simulink model "ADAC_AEBS_FailOperationTest_A2_cs"  (Simulink 7.6)
settings: Solver=ode5  SolverMode=SingleTasking  StartTime=0.0  StopTime=inf  FixedStep=1/100  RelTol=1e-3
PreLoadFcn:
  | check_NUTS_defined;
  | 
  | assignin('base',['model_closed_' bdroot],false);addpath('../includes_AEBS');
InitFcn:
  | PreScanExperimentInitFcn(bdroot)
StopFcn:
  | PreScanExperimentStopFcn(bdroot)
undefined symbols (not defined in the file): DiscIntNeverNeededParam, x_ini_VRML, y_ini_VRML, z_ini_VRML
libraries: simulink x25, PreScanSimulinkLibrary x12, simulink_extras x8, PreScanUsefulBlocks x5, simulink_need_slupdate x1
(part 4 of 7)

== system ADAC_AEBS_FailOperationTest_A2_cs/VISULightSource_Audi_A8_1/conv_FogLightFrontRight ==
  on_off : Inport
  OffColor : Constant  Value="[51   51   51  255   77   77   77  255  102  102  102  255    0    0    0  255]"
  OnColor : Constant  Value="[51   51   51  255  204  204  204  255  102  102  102  255  510  510  510  255]"
  Switch1 : Switch  Threshold=0.5
  RGBcolor : Outport
  wires:
  OffColor/1 -> Switch1/3  "off"
  OnColor/1 -> Switch1/1  "on"
  on_off/1 -> Switch1/2
  Switch1/1 -> RGBcolor/1

== system ADAC_AEBS_FailOperationTest_A2_cs/VISULightSource_Audi_A8_1/conv_FogLightRearLeft ==
  on_off : Inport
  OffColor : Constant  Value="[51   51   51  255   92    0    0  255  102  102  102  255    0    0    0  255]"
  OnColor : Constant  Value="[51   51   51  255  332   51    0  255  102  102  102  255  583   10    0  255]"
  Switch1 : Switch  Threshold=0.5
  RGBcolor : Outport
  wires:
  OffColor/1 -> Switch1/3  "off"
  OnColor/1 -> Switch1/1  "on"
  on_off/1 -> Switch1/2
  Switch1/1 -> RGBcolor/1

== system ADAC_AEBS_FailOperationTest_A2_cs/VISULightSource_Audi_A8_1/conv_FogLightRearRight ==
  on_off : Inport
  OffColor : Constant  Value="[51   51   51  255   92    0    0  255  102  102  102  255    0    0    0  255]"
  OnColor : Constant  Value="[51   51   51  255  332   51    0  255  102  102  102  255  583   10    0  255]"
  Switch1 : Switch  Threshold=0.5
  RGBcolor : Outport
  wires:
  OffColor/1 -> Switch1/3  "off"
  OnColor/1 -> Switch1/1  "on"
  on_off/1 -> Switch1/2
  Switch1/1 -> RGBcolor/1

== system ADAC_AEBS_FailOperationTest_A2_cs/VISULightSource_Audi_A8_1/conv_IndicatorLightsLeft ==
  on_off : Inport
  OffColor : Constant  Value="[51   51   51  255  138   69    0  255  102  102  102  255    0    0    0  255]"
  OnColor : Constant  Value="[51   51   51  255  255  128    0  255  102  102  102  255  255  191    0  255]"
  Switch1 : Switch  Threshold=0.5
  RGBcolor : Outport
  wires:
  Switch1/1 -> RGBcolor/1
  on_off/1 -> Switch1/2
  OnColor/1 -> Switch1/1  "on"
  OffColor/1 -> Switch1/3  "off"

== system ADAC_AEBS_FailOperationTest_A2_cs/VISULightSource_Audi_A8_1/conv_IndicatorLightsRight ==
  on_off : Inport
  OffColor : Constant  Value="[51   51   51  255  138   69    0  255  102  102  102  255    0    0    0  255]"
  OnColor : Constant  Value="[51   51   51  255  255  128    0  255  102  102  102  255  255  191    0  255]"
  Switch1 : Switch  Threshold=0.5
  RGBcolor : Outport
  wires:
  OffColor/1 -> Switch1/3  "off"
  OnColor/1 -> Switch1/1  "on"
  on_off/1 -> Switch1/2
  Switch1/1 -> RGBcolor/1

== system ADAC_AEBS_FailOperationTest_A2_cs/VISULightSource_Audi_A8_1/conv_MainLightFrontLeft ==
  on_off : Inport
  OffColor : Constant  Value="[26   26   26  255   77   77   77  255  102  102  102  255    0    0    0  255]"
  OnColor : Constant  Value="[51   51   51  255  255  255  255  255  102  102  102  255  683  683  683  255]"
  Switch1 : Switch  Threshold=0.5
  RGBcolor : Outport
  wires:
  OffColor/1 -> Switch1/3  "off"
  OnColor/1 -> Switch1/1  "on"
  on_off/1 -> Switch1/2
  Switch1/1 -> RGBcolor/1

== system ADAC_AEBS_FailOperationTest_A2_cs/VISULightSource_Audi_A8_1/conv_MainLightFrontRight ==
  on_off : Inport
  OffColor : Constant  Value="[26   26   26  255   77   77   77  255  102  102  102  255    0    0    0  255]"
  OnColor : Constant  Value="[51   51   51  255  255  255  255  255  102  102  102  255  683  683  683  255]"
  Switch1 : Switch  Threshold=0.5
  RGBcolor : Outport
  wires:
  OffColor/1 -> Switch1/3  "off"
  OnColor/1 -> Switch1/1  "on"
  on_off/1 -> Switch1/2
  Switch1/1 -> RGBcolor/1

== system ADAC_AEBS_FailOperationTest_A2_cs/VISULightSource_Audi_A8_1/conv_MainLightRearLeft ==
  on_off : Inport
  OffColor : Constant  Value="[51   51   51  255   92    0    0  255  102  102  102  255    0    0    0  255]"
  OnColor : Constant  Value="[51   51   51  255  322   51    0  255  102  102  102  255  255   40    0  255]"
  Switch1 : Switch  Threshold=0.5
  RGBcolor : Outport
  wires:
  OffColor/1 -> Switch1/3  "off"
  OnColor/1 -> Switch1/1  "on"
  on_off/1 -> Switch1/2
  Switch1/1 -> RGBcolor/1

== system ADAC_AEBS_FailOperationTest_A2_cs/VISULightSource_Audi_A8_1/conv_MainLightRearRight ==
  on_off : Inport
  OffColor : Constant  Value="[51   51   51  255   92    0    0  255  102  102  102  255    0    0    0  255]"
  OnColor : Constant  Value="[51   51   51  255  322   51    0  255  102  102  102  255  255   40    0  255]"
  Switch1 : Switch  Threshold=0.5
  RGBcolor : Outport
  wires:
  OffColor/1 -> Switch1/3  "off"
  OnColor/1 -> Switch1/1  "on"
  on_off/1 -> Switch1/2
  Switch1/1 -> RGBcolor/1

== system ADAC_AEBS_FailOperationTest_A2_cs/VISULightSource_Audi_A8_1/visu_BrakeLightLeft_0 ==
  Y : Inport
  Assignment : Assignment  IndexMode=Zero-based  SampleTime=TimeStep  IndexOptions=Starting index (dialog)  Indices=PortIndex  OutputSizes=[1 1]
  Data Store Read : DataStoreRead  DataStoreName=SimCoreActuators  SampleTime=TimeStep
  Data Store Write : DataStoreWrite  DataStoreName=SimCoreActuators
  wires:
  Y/1 -> Assignment/2
  Data Store Read/1 -> Assignment/1
  Assignment/1 -> Data Store Write/1

== system ADAC_AEBS_FailOperationTest_A2_cs/VISULightSource_Audi_A8_1/visu_BrakeLightRight_0 ==
  Y : Inport
  Assignment : Assignment  IndexMode=Zero-based  SampleTime=TimeStep  IndexOptions=Starting index (dialog)  Indices=PortIndex  OutputSizes=[1 1]
  Data Store Read : DataStoreRead  DataStoreName=SimCoreActuators  SampleTime=TimeStep
  Data Store Write : DataStoreWrite  DataStoreName=SimCoreActuators
  wires:
  Y/1 -> Assignment/2
  Data Store Read/1 -> Assignment/1
  Assignment/1 -> Data Store Write/1

== system ADAC_AEBS_FailOperationTest_A2_cs/VISULightSource_Audi_A8_1/visu_FogLightFrontLeft_0 ==
  Y : Inport
  Assignment : Assignment  IndexMode=Zero-based  SampleTime=TimeStep  IndexOptions=Starting index (dialog)  Indices=PortIndex  OutputSizes=[1 1]
  Data Store Read : DataStoreRead  DataStoreName=SimCoreActuators  SampleTime=TimeStep
  Data Store Write : DataStoreWrite  DataStoreName=SimCoreActuators
  wires:
  Y/1 -> Assignment/2
  Data Store Read/1 -> Assignment/1
  Assignment/1 -> Data Store Write/1

== system ADAC_AEBS_FailOperationTest_A2_cs/VISULightSource_Audi_A8_1/visu_FogLightFrontRight_0 ==
  Y : Inport
  Assignment : Assignment  IndexMode=Zero-based  SampleTime=TimeStep  IndexOptions=Starting index (dialog)  Indices=PortIndex  OutputSizes=[1 1]
  Data Store Read : DataStoreRead  DataStoreName=SimCoreActuators  SampleTime=TimeStep
  Data Store Write : DataStoreWrite  DataStoreName=SimCoreActuators
  wires:
  Y/1 -> Assignment/2
  Data Store Read/1 -> Assignment/1
  Assignment/1 -> Data Store Write/1

== system ADAC_AEBS_FailOperationTest_A2_cs/VISULightSource_Audi_A8_1/visu_FogLightRearLeft_0 ==
  Y : Inport
  Assignment : Assignment  IndexMode=Zero-based  SampleTime=TimeStep  IndexOptions=Starting index (dialog)  Indices=PortIndex  OutputSizes=[1 1]
  Data Store Read : DataStoreRead  DataStoreName=SimCoreActuators  SampleTime=TimeStep
  Data Store Write : DataStoreWrite  DataStoreName=SimCoreActuators
  wires:
  Y/1 -> Assignment/2
  Data Store Read/1 -> Assignment/1
  Assignment/1 -> Data Store Write/1

== system ADAC_AEBS_FailOperationTest_A2_cs/VISULightSource_Audi_A8_1/visu_FogLightRearRight_0 ==
  Y : Inport
  Assignment : Assignment  IndexMode=Zero-based  SampleTime=TimeStep  IndexOptions=Starting index (dialog)  Indices=PortIndex  OutputSizes=[1 1]
  Data Store Read : DataStoreRead  DataStoreName=SimCoreActuators  SampleTime=TimeStep
  Data Store Write : DataStoreWrite  DataStoreName=SimCoreActuators
  wires:
  Y/1 -> Assignment/2
  Data Store Read/1 -> Assignment/1
  Assignment/1 -> Data Store Write/1

== system ADAC_AEBS_FailOperationTest_A2_cs/VISULightSource_Audi_A8_1/visu_IndicatorLightsLeft_0 ==
  Y : Inport
  Assignment : Assignment  IndexMode=Zero-based  SampleTime=TimeStep  IndexOptions=Starting index (dialog)  Indices=PortIndex  OutputSizes=[1 1]
  Data Store Read : DataStoreRead  DataStoreName=SimCoreActuators  SampleTime=TimeStep
  Data Store Write : DataStoreWrite  DataStoreName=SimCoreActuators
  wires:
  Assignment/1 -> Data Store Write/1
  Data Store Read/1 -> Assignment/1
  Y/1 -> Assignment/2

== system ADAC_AEBS_FailOperationTest_A2_cs/VISULightSource_Audi_A8_1/visu_IndicatorLightsRight_0 ==
  Y : Inport
  Assignment : Assignment  IndexMode=Zero-based  SampleTime=TimeStep  IndexOptions=Starting index (dialog)  Indices=PortIndex  OutputSizes=[1 1]
  Data Store Read : DataStoreRead  DataStoreName=SimCoreActuators  SampleTime=TimeStep
  Data Store Write : DataStoreWrite  DataStoreName=SimCoreActuators
  wires:
  Y/1 -> Assignment/2
  Data Store Read/1 -> Assignment/1
  Assignment/1 -> Data Store Write/1

== system ADAC_AEBS_FailOperationTest_A2_cs/VISULightSource_Audi_A8_1/visu_MainLightFrontLeft_0 ==
  Y : Inport
  Assignment : Assignment  IndexMode=Zero-based  SampleTime=TimeStep  IndexOptions=Starting index (dialog)  Indices=PortIndex  OutputSizes=[1 1]
  Data Store Read : DataStoreRead  DataStoreName=SimCoreActuators  SampleTime=TimeStep
  Data Store Write : DataStoreWrite  DataStoreName=SimCoreActuators
  wires:
  Y/1 -> Assignment/2
  Data Store Read/1 -> Assignment/1
  Assignment/1 -> Data Store Write/1

== system ADAC_AEBS_FailOperationTest_A2_cs/VISULightSource_Audi_A8_1/visu_MainLightFrontRight_0 ==
  Y : Inport
  Assignment : Assignment  IndexMode=Zero-based  SampleTime=TimeStep  IndexOptions=Starting index (dialog)  Indices=PortIndex  OutputSizes=[1 1]
  Data Store Read : DataStoreRead  DataStoreName=SimCoreActuators  SampleTime=TimeStep
  Data Store Write : DataStoreWrite  DataStoreName=SimCoreActuators
  wires:
  Y/1 -> Assignment/2
  Data Store Read/1 -> Assignment/1
  Assignment/1 -> Data Store Write/1

== system ADAC_AEBS_FailOperationTest_A2_cs/VISULightSource_Audi_A8_1/visu_MainLightRearLeft_0 ==
  Y : Inport
  Assignment : Assignment  IndexMode=Zero-based  SampleTime=TimeStep  IndexOptions=Starting index (dialog)  Indices=PortIndex  OutputSizes=[1 1]
  Data Store Read : DataStoreRead  DataStoreName=SimCoreActuators  SampleTime=TimeStep
  Data Store Write : DataStoreWrite  DataStoreName=SimCoreActuators
  wires:
  Y/1 -> Assignment/2
  Data Store Read/1 -> Assignment/1
  Assignment/1 -> Data Store Write/1

== system ADAC_AEBS_FailOperationTest_A2_cs/VISULightSource_Audi_A8_1/visu_MainLightRearRight_0 ==
  Y : Inport
  Assignment : Assignment  IndexMode=Zero-based  SampleTime=TimeStep  IndexOptions=Starting index (dialog)  Indices=PortIndex  OutputSizes=[1 1]
  Data Store Read : DataStoreRead  DataStoreName=SimCoreActuators  SampleTime=TimeStep
  Data Store Write : DataStoreWrite  DataStoreName=SimCoreActuators
  wires:
  Y/1 -> Assignment/2
  Data Store Read/1 -> Assignment/1
  Assignment/1 -> Data Store Write/1

== system ADAC_AEBS_FailOperationTest_A2_cs/VISULightSource_Citroen_C3_1/conv_BrakeLightLeft ==
  on_off : Inport
  OffColor : Constant  Value="[51   51   51  255   92    0    0  255  102  102  102  255    0    0    0  255]"
  OnColor : Constant  Value="[51   51   51  255  332   51    0  255  102  102  102  255  583   47    0  255]"
  Switch1 : Switch  Threshold=0.5
  RGBcolor : Outport
  wires:
  OffColor/1 -> Switch1/3  "off"
  OnColor/1 -> Switch1/1  "on"
  on_off/1 -> Switch1/2
  Switch1/1 -> RGBcolor/1

== system ADAC_AEBS_FailOperationTest_A2_cs/VISULightSource_Citroen_C3_1/conv_BrakeLightRight ==
  on_off : Inport
  OffColor : Constant  Value="[51   51   51  255   92    0    0  255  102  102  102  255    0    0    0  255]"
  OnColor : Constant  Value="[51   51   51  255  332   51    0  255  102  102  102  255  583   47    0  255]"
  Switch1 : Switch  Threshold=0.5
  RGBcolor : Outport
  wires:
  OffColor/1 -> Switch1/3  "off"
  OnColor/1 -> Switch1/1  "on"
  on_off/1 -> Switch1/2
  Switch1/1 -> RGBcolor/1

== system ADAC_AEBS_FailOperationTest_A2_cs/VISULightSource_Citroen_C3_1/conv_FogLightFrontLeft ==
  on_off : Inport
  OffColor : Constant  Value="[51   51   51  255   77   77   77  255  102  102  102  255    0    0    0  255]"
  OnColor : Constant  Value="[51   51   51  255  204  204  204  255  102  102  102  255  510  510  510  255]"
  Switch1 : Switch  Threshold=0.5
  RGBcolor : Outport
  wires:
  OffColor/1 -> Switch1/3  "off"
  OnColor/1 -> Switch1/1  "on"
  on_off/1 -> Switch1/2
  Switch1/1 -> RGBcolor/1

== system ADAC_AEBS_FailOperationTest_A2_cs/VISULightSource_Citroen_C3_1/conv_FogLightFrontRight ==
  on_off : Inport
  OffColor : Constant  Value="[51   51   51  255   77   77   77  255  102  102  102  255    0    0    0  255]"
  OnColor : Constant  Value="[51   51   51  255  204  204  204  255  102  102  102  255  510  510  510  255]"
  Switch1 : Switch  Threshold=0.5
  RGBcolor : Outport
  wires:
  OffColor/1 -> Switch1/3  "off"
  OnColor/1 -> Switch1/1  "on"
  on_off/1 -> Switch1/2
  Switch1/1 -> RGBcolor/1

== system ADAC_AEBS_FailOperationTest_A2_cs/VISULightSource_Citroen_C3_1/conv_IndicatorLightsLeft ==
  on_off : Inport
  OffColor : Constant  Value="[51   51   51  255  138   69    0  255  102  102  102  255    0    0    0  255]"
  OnColor : Constant  Value="[51   51   51  255  255  128    0  255  102  102  102  255  255  191    0  255]"
  Switch1 : Switch  Threshold=0.5
  RGBcolor : Outport
  wires:
  Switch1/1 -> RGBcolor/1
  on_off/1 -> Switch1/2
  OnColor/1 -> Switch1/1  "on"
  OffColor/1 -> Switch1/3  "off"

== system ADAC_AEBS_FailOperationTest_A2_cs/VISULightSource_Citroen_C3_1/conv_IndicatorLightsRight ==
  on_off : Inport
  OffColor : Constant  Value="[51   51   51  255  138   69    0  255  102  102  102  255    0    0    0  255]"
  OnColor : Constant  Value="[51   51   51  255  255  128    0  255  102  102  102  255  255  191    0  255]"
  Switch1 : Switch  Threshold=0.5
  RGBcolor : Outport
  wires:
  OffColor/1 -> Switch1/3  "off"
  OnColor/1 -> Switch1/1  "on"
  on_off/1 -> Switch1/2
  Switch1/1 -> RGBcolor/1

== system ADAC_AEBS_FailOperationTest_A2_cs/VISULightSource_Citroen_C3_1/conv_MainLightFrontLeft ==
  on_off : Inport
  OffColor : Constant  Value="[26   26   26  255   77   77   77  255  102  102  102  255    0    0    0  255]"
  OnColor : Constant  Value="[51   51   51  255  255  255  255  255  102  102  102  255  683  683  683  255]"
  Switch1 : Switch  Threshold=0.5
  RGBcolor : Outport
  wires:
  OffColor/1 -> Switch1/3  "off"
  OnColor/1 -> Switch1/1  "on"
  on_off/1 -> Switch1/2
  Switch1/1 -> RGBcolor/1

== system ADAC_AEBS_FailOperationTest_A2_cs/VISULightSource_Citroen_C3_1/conv_MainLightFrontRight ==
  on_off : Inport
  OffColor : Constant  Value="[26   26   26  255   77   77   77  255  102  102  102  255    0    0    0  255]"
  OnColor : Constant  Value="[51   51   51  255  255  255  255  255  102  102  102  255  683  683  683  255]"
  Switch1 : Switch  Threshold=0.5
  RGBcolor : Outport
  wires:
  OffColor/1 -> Switch1/3  "off"
  OnColor/1 -> Switch1/1  "on"
  on_off/1 -> Switch1/2
  Switch1/1 -> RGBcolor/1

== system ADAC_AEBS_FailOperationTest_A2_cs/VISULightSource_Citroen_C3_1/conv_MainLightRearLeft ==
  on_off : Inport
  OffColor : Constant  Value="[51   51   51  255   92    0    0  255  102  102  102  255    0    0    0  255]"
  OnColor : Constant  Value="[51   51   51  255  322   51    0  255  102  102  102  255  255   40    0  255]"
  Switch1 : Switch  Threshold=0.5
  RGBcolor : Outport
  wires:
  OffColor/1 -> Switch1/3  "off"
  OnColor/1 -> Switch1/1  "on"
  on_off/1 -> Switch1/2
  Switch1/1 -> RGBcolor/1

== system ADAC_AEBS_FailOperationTest_A2_cs/VISULightSource_Citroen_C3_1/conv_MainLightRearRight ==
  on_off : Inport
  OffColor : Constant  Value="[51   51   51  255   92    0    0  255  102  102  102  255    0    0    0  255]"
  OnColor : Constant  Value="[51   51   51  255  322   51    0  255  102  102  102  255  255   40    0  255]"
  Switch1 : Switch  Threshold=0.5
  RGBcolor : Outport
  wires:
  OffColor/1 -> Switch1/3  "off"
  OnColor/1 -> Switch1/1  "on"
  on_off/1 -> Switch1/2
  Switch1/1 -> RGBcolor/1

== system ADAC_AEBS_FailOperationTest_A2_cs/VISULightSource_Citroen_C3_1/visu_BrakeLightLeft_0 ==
  Y : Inport
  Assignment : Assignment  IndexMode=Zero-based  SampleTime=TimeStep  IndexOptions=Starting index (dialog)  Indices=PortIndex  OutputSizes=[1 1]
  Data Store Read : DataStoreRead  DataStoreName=SimCoreActuators  SampleTime=TimeStep
  Data Store Write : DataStoreWrite  DataStoreName=SimCoreActuators
  wires:
  Y/1 -> Assignment/2
  Data Store Read/1 -> Assignment/1
  Assignment/1 -> Data Store Write/1

== system ADAC_AEBS_FailOperationTest_A2_cs/VISULightSource_Citroen_C3_1/visu_BrakeLightRight_0 ==
  Y : Inport
  Assignment : Assignment  IndexMode=Zero-based  SampleTime=TimeStep  IndexOptions=Starting index (dialog)  Indices=PortIndex  OutputSizes=[1 1]
  Data Store Read : DataStoreRead  DataStoreName=SimCoreActuators  SampleTime=TimeStep
  Data Store Write : DataStoreWrite  DataStoreName=SimCoreActuators
  wires:
  Y/1 -> Assignment/2
  Data Store Read/1 -> Assignment/1
  Assignment/1 -> Data Store Write/1

== system ADAC_AEBS_FailOperationTest_A2_cs/VISULightSource_Citroen_C3_1/visu_FogLightFrontLeft_0 ==
  Y : Inport
  Assignment : Assignment  IndexMode=Zero-based  SampleTime=TimeStep  IndexOptions=Starting index (dialog)  Indices=PortIndex  OutputSizes=[1 1]
  Data Store Read : DataStoreRead  DataStoreName=SimCoreActuators  SampleTime=TimeStep
  Data Store Write : DataStoreWrite  DataStoreName=SimCoreActuators
  wires:
  Y/1 -> Assignment/2
  Data Store Read/1 -> Assignment/1
  Assignment/1 -> Data Store Write/1

== system ADAC_AEBS_FailOperationTest_A2_cs/VISULightSource_Citroen_C3_1/visu_FogLightFrontRight_0 ==
  Y : Inport
  Assignment : Assignment  IndexMode=Zero-based  SampleTime=TimeStep  IndexOptions=Starting index (dialog)  Indices=PortIndex  OutputSizes=[1 1]
  Data Store Read : DataStoreRead  DataStoreName=SimCoreActuators  SampleTime=TimeStep
  Data Store Write : DataStoreWrite  DataStoreName=SimCoreActuators
  wires:
  Y/1 -> Assignment/2
  Data Store Read/1 -> Assignment/1
  Assignment/1 -> Data Store Write/1

== system ADAC_AEBS_FailOperationTest_A2_cs/VISULightSource_Citroen_C3_1/visu_IndicatorLightsLeft_0 ==
  Y : Inport
  Assignment : Assignment  IndexMode=Zero-based  SampleTime=TimeStep  IndexOptions=Starting index (dialog)  Indices=PortIndex  OutputSizes=[1 1]
  Data Store Read : DataStoreRead  DataStoreName=SimCoreActuators  SampleTime=TimeStep
  Data Store Write : DataStoreWrite  DataStoreName=SimCoreActuators
  wires:
  Assignment/1 -> Data Store Write/1
  Data Store Read/1 -> Assignment/1
  Y/1 -> Assignment/2

== system ADAC_AEBS_FailOperationTest_A2_cs/VISULightSource_Citroen_C3_1/visu_IndicatorLightsRight_0 ==
  Y : Inport
  Assignment : Assignment  IndexMode=Zero-based  SampleTime=TimeStep  IndexOptions=Starting index (dialog)  Indices=PortIndex  OutputSizes=[1 1]
  Data Store Read : DataStoreRead  DataStoreName=SimCoreActuators  SampleTime=TimeStep
  Data Store Write : DataStoreWrite  DataStoreName=SimCoreActuators
  wires:
  Y/1 -> Assignment/2
  Data Store Read/1 -> Assignment/1
  Assignment/1 -> Data Store Write/1

== system ADAC_AEBS_FailOperationTest_A2_cs/VISULightSource_Citroen_C3_1/visu_MainLightFrontLeft_0 ==
  Y : Inport
  Assignment : Assignment  IndexMode=Zero-based  SampleTime=TimeStep  IndexOptions=Starting index (dialog)  Indices=PortIndex  OutputSizes=[1 1]
  Data Store Read : DataStoreRead  DataStoreName=SimCoreActuators  SampleTime=TimeStep
  Data Store Write : DataStoreWrite  DataStoreName=SimCoreActuators
  wires:
  Y/1 -> Assignment/2
  Data Store Read/1 -> Assignment/1
  Assignment/1 -> Data Store Write/1

== system ADAC_AEBS_FailOperationTest_A2_cs/VISULightSource_Citroen_C3_1/visu_MainLightFrontRight_0 ==
  Y : Inport
  Assignment : Assignment  IndexMode=Zero-based  SampleTime=TimeStep  IndexOptions=Starting index (dialog)  Indices=PortIndex  OutputSizes=[1 1]
  Data Store Read : DataStoreRead  DataStoreName=SimCoreActuators  SampleTime=TimeStep
  Data Store Write : DataStoreWrite  DataStoreName=SimCoreActuators
  wires:
  Y/1 -> Assignment/2
  Data Store Read/1 -> Assignment/1
  Assignment/1 -> Data Store Write/1

== system ADAC_AEBS_FailOperationTest_A2_cs/VISULightSource_Citroen_C3_1/visu_MainLightRearLeft_0 ==
  Y : Inport
  Assignment : Assignment  IndexMode=Zero-based  SampleTime=TimeStep  IndexOptions=Starting index (dialog)  Indices=PortIndex  OutputSizes=[1 1]
  Data Store Read : DataStoreRead  DataStoreName=SimCoreActuators  SampleTime=TimeStep
  Data Store Write : DataStoreWrite  DataStoreName=SimCoreActuators
  wires:
  Y/1 -> Assignment/2
  Data Store Read/1 -> Assignment/1
  Assignment/1 -> Data Store Write/1

== system ADAC_AEBS_FailOperationTest_A2_cs/VISULightSource_Citroen_C3_1/visu_MainLightRearRight_0 ==
  Y : Inport
  Assignment : Assignment  IndexMode=Zero-based  SampleTime=TimeStep  IndexOptions=Starting index (dialog)  Indices=PortIndex  OutputSizes=[1 1]
  Data Store Read : DataStoreRead  DataStoreName=SimCoreActuators  SampleTime=TimeStep
  Data Store Write : DataStoreWrite  DataStoreName=SimCoreActuators
  wires:
  Y/1 -> Assignment/2
  Data Store Read/1 -> Assignment/1
  Assignment/1 -> Data Store Write/1

== system ADAC_AEBS_FailOperationTest_A2_cs/VISUSteer_Audi_A8_1/conv_SteeringColumn ==
  angle [deg] : Inport
  Constant13 : Constant  Value=[0 1 0]
  Mux8 : Mux  Inputs=2
  deg2rad : Gain  Gain=pi/180
  QuaternionVisu [rad] : Outport
  wires:
  deg2rad/1 -> Mux8/2
  Constant13/1 -> Mux8/1
  Mux8/1 -> QuaternionVisu [rad]/1
  angle [deg]/1 -> deg2rad/1

== system ADAC_AEBS_FailOperationTest_A2_cs/VISUSteer_Audi_A8_1/conv_SteeringWheel ==
  angle [deg] : Inport
  Constant13 : Constant  Value=[-1 0 0]
  Mux8 : Mux  Inputs=2
  deg2rad : Gain  Gain=pi/180
  QuaternionVisu [rad] : Outport
  wires:
  deg2rad/1 -> Mux8/2
  Constant13/1 -> Mux8/1
  Mux8/1 -> QuaternionVisu [rad]/1
  angle [deg]/1 -> deg2rad/1

== system ADAC_AEBS_FailOperationTest_A2_cs/VISUSteer_Audi_A8_1/visu_SteeringColumn ==
  Y : Inport
  Assignment : Assignment  IndexMode=Zero-based  SampleTime=TimeStep  IndexOptions=Starting index (dialog)  Indices=PortIndex  OutputSizes=[1 1]
  Data Store Read : DataStoreRead  DataStoreName=SimCoreActuators  SampleTime=TimeStep
  Data Store Write : DataStoreWrite  DataStoreName=SimCoreActuators
  wires:
  Assignment/1 -> Data Store Write/1
  Data Store Read/1 -> Assignment/1
  Y/1 -> Assignment/2

== system ADAC_AEBS_FailOperationTest_A2_cs/VISUSteer_Audi_A8_1/visu_SteeringWheel ==
  Y : Inport
  Assignment : Assignment  IndexMode=Zero-based  SampleTime=TimeStep  IndexOptions=Starting index (dialog)  Indices=PortIndex  OutputSizes=[1 1]
  Data Store Read : DataStoreRead  DataStoreName=SimCoreActuators  SampleTime=TimeStep
  Data Store Write : DataStoreWrite  DataStoreName=SimCoreActuators
  wires:
  Assignment/1 -> Data Store Write/1
  Data Store Read/1 -> Assignment/1
  Y/1 -> Assignment/2

== system ADAC_AEBS_FailOperationTest_A2_cs/VISUSteer_Citroen_C3_1/conv_SteeringColumn ==
  angle [deg] : Inport
  Constant13 : Constant  Value=[0 1 0]
  Mux8 : Mux  Inputs=2
  deg2rad : Gain  Gain=pi/180
  QuaternionVisu [rad] : Outport
  wires:
  deg2rad/1 -> Mux8/2
  Constant13/1 -> Mux8/1
  Mux8/1 -> QuaternionVisu [rad]/1
  angle [deg]/1 -> deg2rad/1

== system ADAC_AEBS_FailOperationTest_A2_cs/VISUSteer_Citroen_C3_1/conv_SteeringWheel ==
  angle [deg] : Inport
  Constant13 : Constant  Value=[-1 0 0]
  Mux8 : Mux  Inputs=2
  deg2rad : Gain  Gain=pi/180
  QuaternionVisu [rad] : Outport
  wires:
  deg2rad/1 -> Mux8/2
  Constant13/1 -> Mux8/1
  Mux8/1 -> QuaternionVisu [rad]/1
  angle [deg]/1 -> deg2rad/1

== system ADAC_AEBS_FailOperationTest_A2_cs/VISUSteer_Citroen_C3_1/visu_SteeringColumn ==
  Y : Inport
  Assignment : Assignment  IndexMode=Zero-based  SampleTime=TimeStep  IndexOptions=Starting index (dialog)  Indices=PortIndex  OutputSizes=[1 1]
  Data Store Read : DataStoreRead  DataStoreName=SimCoreActuators  SampleTime=TimeStep
  Data Store Write : DataStoreWrite  DataStoreName=SimCoreActuators
  wires:
  Assignment/1 -> Data Store Write/1
  Data Store Read/1 -> Assignment/1
  Y/1 -> Assignment/2

== system ADAC_AEBS_FailOperationTest_A2_cs/VISUSteer_Citroen_C3_1/visu_SteeringWheel ==
  Y : Inport
  Assignment : Assignment  IndexMode=Zero-based  SampleTime=TimeStep  IndexOptions=Starting index (dialog)  Indices=PortIndex  OutputSizes=[1 1]
  Data Store Read : DataStoreRead  DataStoreName=SimCoreActuators  SampleTime=TimeStep
  Data Store Write : DataStoreWrite  DataStoreName=SimCoreActuators
  wires:
  Assignment/1 -> Data Store Write/1
  Data Store Read/1 -> Assignment/1
  Y/1 -> Assignment/2

== system ADAC_AEBS_FailOperationTest_A2_cs/VISUWheels_Audi_A8_1/conv_RotWheelFL ==
  BryantISO [deg] : Inport
  Fcn10 : Fcn  Expr=cos(u(1))*sin(u(3))+sin(u(1))*sin(u(2))*cos(u(3))
  Fcn11 : Fcn  Expr=sin(u(1))*sin(u(3))-cos(u(1))*sin(u(2))*cos(u(3))
  Fcn12 : Fcn  Expr=-cos(u(2))*sin(u(3))
  Fcn13 : Fcn  Expr=cos(u(1))*cos(u(3))-sin(u(1))*sin(u(2))*sin(u(3))
  Fcn14 : Fcn  Expr=sin(u(1))*cos(u(3))+cos(u(1))*sin(u(2))*sin(u(3))
  Fcn15 : Fcn  Expr=sin(u(2))
  Fcn16 : Fcn  Expr=-sin(u(1))*cos(u(2))
  Fcn17 : Fcn  Expr=cos(u(1))*cos(u(2))
  Fcn9 : Fcn  Expr=cos(u(2))*cos(u(3))
  Mux1 : Mux  Inputs=9
  RotMat2AxisAngle : Subsystem
  deg2rad : Gain  Gain=pi/180
  xyz 2 zxy : Selector  InputPortWidth=3  IndexOptions=Index vector (dialog)  Indices=[3 1 2]  OutputSizes=1
  zxy 2 xyz : Selector  InputPortWidth=4  IndexOptions=Index vector (dialog)  Indices=[2 3 1 4]  OutputSizes=1
  QuaternionVisu [rad] : Outport
  wires:
  zxy 2 xyz/1 -> QuaternionVisu [rad]/1
  xyz 2 zxy/1 -> deg2rad/1
  deg2rad/1 -> Fcn17/1, Fcn16/1, Fcn15/1, Fcn14/1, Fcn13/1, Fcn12/1, Fcn11/1, Fcn10/1, Fcn9/1
  BryantISO [deg]/1 -> xyz 2 zxy/1  "BryantAngles rotx roty rotz Visu"
  RotMat2AxisAngle/1(Angles_Visu) -> zxy 2 xyz/1
  Mux1/1 -> RotMat2AxisAngle/1(RotMat_Visu)  "RotationMatrix Visu"
  Fcn17/1 -> Mux1/9
  Fcn16/1 -> Mux1/8
  Fcn15/1 -> Mux1/7
  Fcn14/1 -> Mux1/6
  Fcn13/1 -> Mux1/5
  Fcn12/1 -> Mux1/4
  Fcn11/1 -> Mux1/3
  Fcn10/1 -> Mux1/2
  Fcn9/1 -> Mux1/1

== system ADAC_AEBS_FailOperationTest_A2_cs/VISUWheels_Audi_A8_1/conv_RotWheelFR ==
  BryantISO [deg] : Inport
  Fcn10 : Fcn  Expr=cos(u(1))*sin(u(3))+sin(u(1))*sin(u(2))*cos(u(3))
  Fcn11 : Fcn  Expr=sin(u(1))*sin(u(3))-cos(u(1))*sin(u(2))*cos(u(3))
  Fcn12 : Fcn  Expr=-cos(u(2))*sin(u(3))
  Fcn13 : Fcn  Expr=cos(u(1))*cos(u(3))-sin(u(1))*sin(u(2))*sin(u(3))
  Fcn14 : Fcn  Expr=sin(u(1))*cos(u(3))+cos(u(1))*sin(u(2))*sin(u(3))
  Fcn15 : Fcn  Expr=sin(u(2))
  Fcn16 : Fcn  Expr=-sin(u(1))*cos(u(2))
  Fcn17 : Fcn  Expr=cos(u(1))*cos(u(2))
  Fcn9 : Fcn  Expr=cos(u(2))*cos(u(3))
  Mux1 : Mux  Inputs=9
  RotMat2AxisAngle : Subsystem
  deg2rad : Gain  Gain=pi/180
  xyz 2 zxy : Selector  InputPortWidth=3  IndexOptions=Index vector (dialog)  Indices=[3 1 2]  OutputSizes=1
  zxy 2 xyz : Selector  InputPortWidth=4  IndexOptions=Index vector (dialog)  Indices=[2 3 1 4]  OutputSizes=1
  QuaternionVisu [rad] : Outport
  wires:
  zxy 2 xyz/1 -> QuaternionVisu [rad]/1
  xyz 2 zxy/1 -> deg2rad/1
  deg2rad/1 -> Fcn17/1, Fcn16/1, Fcn15/1, Fcn14/1, Fcn13/1, Fcn12/1, Fcn11/1, Fcn10/1, Fcn9/1
  BryantISO [deg]/1 -> xyz 2 zxy/1  "BryantAngles rotx roty rotz Visu"
  RotMat2AxisAngle/1(Angles_Visu) -> zxy 2 xyz/1
  Mux1/1 -> RotMat2AxisAngle/1(RotMat_Visu)  "RotationMatrix Visu"
  Fcn17/1 -> Mux1/9
  Fcn16/1 -> Mux1/8
  Fcn15/1 -> Mux1/7
  Fcn14/1 -> Mux1/6
  Fcn13/1 -> Mux1/5
  Fcn12/1 -> Mux1/4
  Fcn11/1 -> Mux1/3
  Fcn10/1 -> Mux1/2
  Fcn9/1 -> Mux1/1

== system ADAC_AEBS_FailOperationTest_A2_cs/VISUWheels_Audi_A8_1/conv_RotWheelRL ==
  BryantISO [deg] : Inport
  Fcn10 : Fcn  Expr=cos(u(1))*sin(u(3))+sin(u(1))*sin(u(2))*cos(u(3))
  Fcn11 : Fcn  Expr=sin(u(1))*sin(u(3))-cos(u(1))*sin(u(2))*cos(u(3))
  Fcn12 : Fcn  Expr=-cos(u(2))*sin(u(3))
  Fcn13 : Fcn  Expr=cos(u(1))*cos(u(3))-sin(u(1))*sin(u(2))*sin(u(3))
  Fcn14 : Fcn  Expr=sin(u(1))*cos(u(3))+cos(u(1))*sin(u(2))*sin(u(3))
  Fcn15 : Fcn  Expr=sin(u(2))
  Fcn16 : Fcn  Expr=-sin(u(1))*cos(u(2))
  Fcn17 : Fcn  Expr=cos(u(1))*cos(u(2))
  Fcn9 : Fcn  Expr=cos(u(2))*cos(u(3))
  Mux1 : Mux  Inputs=9
  RotMat2AxisAngle : Subsystem
  deg2rad : Gain  Gain=pi/180
  xyz 2 zxy : Selector  InputPortWidth=3  IndexOptions=Index vector (dialog)  Indices=[3 1 2]  OutputSizes=1
  zxy 2 xyz : Selector  InputPortWidth=4  IndexOptions=Index vector (dialog)  Indices=[2 3 1 4]  OutputSizes=1
  QuaternionVisu [rad] : Outport
  wires:
  zxy 2 xyz/1 -> QuaternionVisu [rad]/1
  xyz 2 zxy/1 -> deg2rad/1
  deg2rad/1 -> Fcn17/1, Fcn16/1, Fcn15/1, Fcn14/1, Fcn13/1, Fcn12/1, Fcn11/1, Fcn10/1, Fcn9/1
  BryantISO [deg]/1 -> xyz 2 zxy/1  "BryantAngles rotx roty rotz Visu"
  RotMat2AxisAngle/1(Angles_Visu) -> zxy 2 xyz/1
  Mux1/1 -> RotMat2AxisAngle/1(RotMat_Visu)  "RotationMatrix Visu"
  Fcn17/1 -> Mux1/9
  Fcn16/1 -> Mux1/8
  Fcn15/1 -> Mux1/7
  Fcn14/1 -> Mux1/6
  Fcn13/1 -> Mux1/5
  Fcn12/1 -> Mux1/4
  Fcn11/1 -> Mux1/3
  Fcn10/1 -> Mux1/2
  Fcn9/1 -> Mux1/1

== system ADAC_AEBS_FailOperationTest_A2_cs/VISUWheels_Audi_A8_1/conv_RotWheelRR ==
  BryantISO [deg] : Inport
  Fcn10 : Fcn  Expr=cos(u(1))*sin(u(3))+sin(u(1))*sin(u(2))*cos(u(3))
  Fcn11 : Fcn  Expr=sin(u(1))*sin(u(3))-cos(u(1))*sin(u(2))*cos(u(3))
  Fcn12 : Fcn  Expr=-cos(u(2))*sin(u(3))
  Fcn13 : Fcn  Expr=cos(u(1))*cos(u(3))-sin(u(1))*sin(u(2))*sin(u(3))
  Fcn14 : Fcn  Expr=sin(u(1))*cos(u(3))+cos(u(1))*sin(u(2))*sin(u(3))
  Fcn15 : Fcn  Expr=sin(u(2))
  Fcn16 : Fcn  Expr=-sin(u(1))*cos(u(2))
  Fcn17 : Fcn  Expr=cos(u(1))*cos(u(2))
  Fcn9 : Fcn  Expr=cos(u(2))*cos(u(3))
  Mux1 : Mux  Inputs=9
  RotMat2AxisAngle : Subsystem
  deg2rad : Gain  Gain=pi/180
  xyz 2 zxy : Selector  InputPortWidth=3  IndexOptions=Index vector (dialog)  Indices=[3 1 2]  OutputSizes=1
  zxy 2 xyz : Selector  InputPortWidth=4  IndexOptions=Index vector (dialog)  Indices=[2 3 1 4]  OutputSizes=1
  QuaternionVisu [rad] : Outport
  wires:
  zxy 2 xyz/1 -> QuaternionVisu [rad]/1
  xyz 2 zxy/1 -> deg2rad/1
  deg2rad/1 -> Fcn17/1, Fcn16/1, Fcn15/1, Fcn14/1, Fcn13/1, Fcn12/1, Fcn11/1, Fcn10/1, Fcn9/1
  BryantISO [deg]/1 -> xyz 2 zxy/1  "BryantAngles rotx roty rotz Visu"
  RotMat2AxisAngle/1(Angles_Visu) -> zxy 2 xyz/1
  Mux1/1 -> RotMat2AxisAngle/1(RotMat_Visu)  "RotationMatrix Visu"
  Fcn17/1 -> Mux1/9
  Fcn16/1 -> Mux1/8
  Fcn15/1 -> Mux1/7
  Fcn14/1 -> Mux1/6
  Fcn13/1 -> Mux1/5
  Fcn12/1 -> Mux1/4
  Fcn11/1 -> Mux1/3
  Fcn10/1 -> Mux1/2
  Fcn9/1 -> Mux1/1

== system ADAC_AEBS_FailOperationTest_A2_cs/VISUWheels_Audi_A8_1/conv_TransWheelFL ==
  transISO [m] : Inport
  Gain1 : Gain  Gain=Gain_xISO
  Gain2 : Gain  Gain=Gain_yISO
  Gain3 : Gain  Gain=Gain_zISO
  Mux2 : Mux  Inputs=3
  Sum : Sum  Inputs=|++
  pos_ini_Visu : Subsystem
  transISO2Visu : Subsystem
  transVisu [m] : Outport
  wires:
  Gain3/1 -> Mux2/3
  Gain2/1 -> Mux2/2
  Gain1/1 -> Mux2/1
  Sum/1 -> transVisu [m]/1
  pos_ini_Visu/1(pos_ini_Visu) -> Sum/2
  Mux2/1 -> Sum/1
  transISO [m]/1 -> transISO2Visu/1(transISO)
  transISO2Visu/1(trans_x_Visu) -> Gain1/1
  transISO2Visu/2(trans_y_Visu) -> Gain2/1
  transISO2Visu/3(trans_z_Visu) -> Gain3/1

== system ADAC_AEBS_FailOperationTest_A2_cs/VISUWheels_Audi_A8_1/conv_TransWheelFR ==
  transISO [m] : Inport
  Gain1 : Gain  Gain=Gain_xISO
  Gain2 : Gain  Gain=Gain_yISO
  Gain3 : Gain  Gain=Gain_zISO
  Mux2 : Mux  Inputs=3
  Sum : Sum  Inputs=|++
  pos_ini_Visu : Subsystem
  transISO2Visu : Subsystem
  transVisu [m] : Outport
  wires:
  Gain3/1 -> Mux2/3
  Gain2/1 -> Mux2/2
  Gain1/1 -> Mux2/1
  Sum/1 -> transVisu [m]/1
  pos_ini_Visu/1(pos_ini_Visu) -> Sum/2
  Mux2/1 -> Sum/1
  transISO [m]/1 -> transISO2Visu/1(transISO)
  transISO2Visu/1(trans_x_Visu) -> Gain1/1
  transISO2Visu/2(trans_y_Visu) -> Gain2/1
  transISO2Visu/3(trans_z_Visu) -> Gain3/1

== system ADAC_AEBS_FailOperationTest_A2_cs/VISUWheels_Audi_A8_1/conv_TransWheelRL ==
  transISO [m] : Inport
  Gain1 : Gain  Gain=Gain_xISO
  Gain2 : Gain  Gain=Gain_yISO
  Gain3 : Gain  Gain=Gain_zISO
  Mux2 : Mux  Inputs=3
  Sum : Sum  Inputs=|++
  pos_ini_Visu : Subsystem
  transISO2Visu : Subsystem
  transVisu [m] : Outport
  wires:
  Gain3/1 -> Mux2/3
  Gain2/1 -> Mux2/2
  Gain1/1 -> Mux2/1
  Sum/1 -> transVisu [m]/1
  pos_ini_Visu/1(pos_ini_Visu) -> Sum/2
  Mux2/1 -> Sum/1
  transISO2Visu/3(trans_z_Visu) -> Gain3/1
  transISO2Visu/2(trans_y_Visu) -> Gain2/1
  transISO [m]/1 -> transISO2Visu/1(transISO)
  transISO2Visu/1(trans_x_Visu) -> Gain1/1

== system ADAC_AEBS_FailOperationTest_A2_cs/VISUWheels_Audi_A8_1/conv_TransWheelRR ==
  transISO [m] : Inport
  Gain1 : Gain  Gain=Gain_xISO
  Gain2 : Gain  Gain=Gain_yISO
  Gain3 : Gain  Gain=Gain_zISO
  Mux2 : Mux  Inputs=3
  Sum : Sum  Inputs=|++
  pos_ini_Visu : Subsystem
  transISO2Visu : Subsystem
  transVisu [m] : Outport
  wires:
  Gain3/1 -> Mux2/3
  Gain2/1 -> Mux2/2
  Gain1/1 -> Mux2/1
  Sum/1 -> transVisu [m]/1
  pos_ini_Visu/1(pos_ini_Visu) -> Sum/2
  Mux2/1 -> Sum/1
  transISO2Visu/3(trans_z_Visu) -> Gain3/1
  transISO2Visu/2(trans_y_Visu) -> Gain2/1
  transISO [m]/1 -> transISO2Visu/1(transISO)
  transISO2Visu/1(trans_x_Visu) -> Gain1/1

== system ADAC_AEBS_FailOperationTest_A2_cs/VISUWheels_Audi_A8_1/visu_RotWheelFL ==
  Y : Inport
  Assignment : Assignment  IndexMode=Zero-based  SampleTime=TimeStep  IndexOptions=Starting index (dialog)  Indices=PortIndex  OutputSizes=[1 1]
  Data Store Read : DataStoreRead  DataStoreName=SimCoreActuators  SampleTime=TimeStep
  Data Store Write : DataStoreWrite  DataStoreName=SimCoreActuators
  wires:
  Y/1 -> Assignment/2
  Data Store Read/1 -> Assignment/1
  Assignment/1 -> Data Store Write/1

== system ADAC_AEBS_FailOperationTest_A2_cs/VISUWheels_Audi_A8_1/visu_RotWheelFR ==
  Y : Inport
  Assignment : Assignment  IndexMode=Zero-based  SampleTime=TimeStep  IndexOptions=Starting index (dialog)  Indices=PortIndex  OutputSizes=[1 1]
  Data Store Read : DataStoreRead  DataStoreName=SimCoreActuators  SampleTime=TimeStep
  Data Store Write : DataStoreWrite  DataStoreName=SimCoreActuators
  wires:
  Y/1 -> Assignment/2
  Data Store Read/1 -> Assignment/1
  Assignment/1 -> Data Store Write/1

== system ADAC_AEBS_FailOperationTest_A2_cs/VISUWheels_Audi_A8_1/visu_RotWheelRL ==
  Y : Inport
  Assignment : Assignment  IndexMode=Zero-based  SampleTime=TimeStep  IndexOptions=Starting index (dialog)  Indices=PortIndex  OutputSizes=[1 1]
  Data Store Read : DataStoreRead  DataStoreName=SimCoreActuators  SampleTime=TimeStep
  Data Store Write : DataStoreWrite  DataStoreName=SimCoreActuators
  wires:
  Y/1 -> Assignment/2
  Data Store Read/1 -> Assignment/1
  Assignment/1 -> Data Store Write/1

== system ADAC_AEBS_FailOperationTest_A2_cs/VISUWheels_Audi_A8_1/visu_RotWheelRR ==
  Y : Inport
  Assignment : Assignment  IndexMode=Zero-based  SampleTime=TimeStep  IndexOptions=Starting index (dialog)  Indices=PortIndex  OutputSizes=[1 1]
  Data Store Read : DataStoreRead  DataStoreName=SimCoreActuators  SampleTime=TimeStep
  Data Store Write : DataStoreWrite  DataStoreName=SimCoreActuators
  wires:
  Y/1 -> Assignment/2
  Data Store Read/1 -> Assignment/1
  Assignment/1 -> Data Store Write/1

== system ADAC_AEBS_FailOperationTest_A2_cs/VISUWheels_Audi_A8_1/visu_TransWheelFL ==
  Y : Inport
  Assignment : Assignment  IndexMode=Zero-based  SampleTime=TimeStep  IndexOptions=Starting index (dialog)  Indices=PortIndex  OutputSizes=[1 1]
  Data Store Read : DataStoreRead  DataStoreName=SimCoreActuators  SampleTime=TimeStep
  Data Store Write : DataStoreWrite  DataStoreName=SimCoreActuators
  wires:
  Y/1 -> Assignment/2
  Data Store Read/1 -> Assignment/1
  Assignment/1 -> Data Store Write/1

== system ADAC_AEBS_FailOperationTest_A2_cs/VISUWheels_Audi_A8_1/visu_TransWheelFR ==
  Y : Inport
  Assignment : Assignment  IndexMode=Zero-based  SampleTime=TimeStep  IndexOptions=Starting index (dialog)  Indices=PortIndex  OutputSizes=[1 1]
  Data Store Read : DataStoreRead  DataStoreName=SimCoreActuators  SampleTime=TimeStep
  Data Store Write : DataStoreWrite  DataStoreName=SimCoreActuators
  wires:
  Y/1 -> Assignment/2
  Data Store Read/1 -> Assignment/1
  Assignment/1 -> Data Store Write/1

== system ADAC_AEBS_FailOperationTest_A2_cs/VISUWheels_Audi_A8_1/visu_TransWheelRL ==
  Y : Inport
  Assignment : Assignment  IndexMode=Zero-based  SampleTime=TimeStep  IndexOptions=Starting index (dialog)  Indices=PortIndex  OutputSizes=[1 1]
  Data Store Read : DataStoreRead  DataStoreName=SimCoreActuators  SampleTime=TimeStep
  Data Store Write : DataStoreWrite  DataStoreName=SimCoreActuators
  wires:
  Y/1 -> Assignment/2
  Data Store Read/1 -> Assignment/1
  Assignment/1 -> Data Store Write/1

== system ADAC_AEBS_FailOperationTest_A2_cs/VISUWheels_Audi_A8_1/visu_TransWheelRR ==
  Y : Inport
  Assignment : Assignment  IndexMode=Zero-based  SampleTime=TimeStep  IndexOptions=Starting index (dialog)  Indices=PortIndex  OutputSizes=[1 1]
  Data Store Read : DataStoreRead  DataStoreName=SimCoreActuators  SampleTime=TimeStep
  Data Store Write : DataStoreWrite  DataStoreName=SimCoreActuators
  wires:
  Y/1 -> Assignment/2
  Data Store Read/1 -> Assignment/1
  Assignment/1 -> Data Store Write/1

== system ADAC_AEBS_FailOperationTest_A2_cs/VISUWheels_Citroen_C3_1/conv_RotWheelFL ==
  BryantISO [deg] : Inport
  Fcn10 : Fcn  Expr=cos(u(1))*sin(u(3))+sin(u(1))*sin(u(2))*cos(u(3))
  Fcn11 : Fcn  Expr=sin(u(1))*sin(u(3))-cos(u(1))*sin(u(2))*cos(u(3))
  Fcn12 : Fcn  Expr=-cos(u(2))*sin(u(3))
  Fcn13 : Fcn  Expr=cos(u(1))*cos(u(3))-sin(u(1))*sin(u(2))*sin(u(3))
  Fcn14 : Fcn  Expr=sin(u(1))*cos(u(3))+cos(u(1))*sin(u(2))*sin(u(3))
  Fcn15 : Fcn  Expr=sin(u(2))
  Fcn16 : Fcn  Expr=-sin(u(1))*cos(u(2))
  Fcn17 : Fcn  Expr=cos(u(1))*cos(u(2))
  Fcn9 : Fcn  Expr=cos(u(2))*cos(u(3))
  Mux1 : Mux  Inputs=9
  RotMat2AxisAngle : Subsystem
  deg2rad : Gain  Gain=pi/180
  xyz 2 zxy : Selector  InputPortWidth=3  IndexOptions=Index vector (dialog)  Indices=[3 1 2]  OutputSizes=1
  zxy 2 xyz : Selector  InputPortWidth=4  IndexOptions=Index vector (dialog)  Indices=[2 3 1 4]  OutputSizes=1
  QuaternionVisu [rad] : Outport
  wires:
  zxy 2 xyz/1 -> QuaternionVisu [rad]/1
  xyz 2 zxy/1 -> deg2rad/1
  deg2rad/1 -> Fcn17/1, Fcn16/1, Fcn15/1, Fcn14/1, Fcn13/1, Fcn12/1, Fcn11/1, Fcn10/1, Fcn9/1
  BryantISO [deg]/1 -> xyz 2 zxy/1  "BryantAngles rotx roty rotz Visu"
  RotMat2AxisAngle/1(Angles_Visu) -> zxy 2 xyz/1
  Mux1/1 -> RotMat2AxisAngle/1(RotMat_Visu)  "RotationMatrix Visu"
  Fcn17/1 -> Mux1/9
  Fcn16/1 -> Mux1/8
  Fcn15/1 -> Mux1/7
  Fcn14/1 -> Mux1/6
  Fcn13/1 -> Mux1/5
  Fcn12/1 -> Mux1/4
  Fcn11/1 -> Mux1/3
  Fcn10/1 -> Mux1/2
  Fcn9/1 -> Mux1/1

== system ADAC_AEBS_FailOperationTest_A2_cs/VISUWheels_Citroen_C3_1/conv_RotWheelFR ==
  BryantISO [deg] : Inport
  Fcn10 : Fcn  Expr=cos(u(1))*sin(u(3))+sin(u(1))*sin(u(2))*cos(u(3))
  Fcn11 : Fcn  Expr=sin(u(1))*sin(u(3))-cos(u(1))*sin(u(2))*cos(u(3))
  Fcn12 : Fcn  Expr=-cos(u(2))*sin(u(3))
  Fcn13 : Fcn  Expr=cos(u(1))*cos(u(3))-sin(u(1))*sin(u(2))*sin(u(3))
  Fcn14 : Fcn  Expr=sin(u(1))*cos(u(3))+cos(u(1))*sin(u(2))*sin(u(3))
  Fcn15 : Fcn  Expr=sin(u(2))
  Fcn16 : Fcn  Expr=-sin(u(1))*cos(u(2))
  Fcn17 : Fcn  Expr=cos(u(1))*cos(u(2))
  Fcn9 : Fcn  Expr=cos(u(2))*cos(u(3))
  Mux1 : Mux  Inputs=9
  RotMat2AxisAngle : Subsystem
  deg2rad : Gain  Gain=pi/180
  xyz 2 zxy : Selector  InputPortWidth=3  IndexOptions=Index vector (dialog)  Indices=[3 1 2]  OutputSizes=1
  zxy 2 xyz : Selector  InputPortWidth=4  IndexOptions=Index vector (dialog)  Indices=[2 3 1 4]  OutputSizes=1
  QuaternionVisu [rad] : Outport
  wires:
  zxy 2 xyz/1 -> QuaternionVisu [rad]/1
  xyz 2 zxy/1 -> deg2rad/1
  deg2rad/1 -> Fcn17/1, Fcn16/1, Fcn15/1, Fcn14/1, Fcn13/1, Fcn12/1, Fcn11/1, Fcn10/1, Fcn9/1
  BryantISO [deg]/1 -> xyz 2 zxy/1  "BryantAngles rotx roty rotz Visu"
  RotMat2AxisAngle/1(Angles_Visu) -> zxy 2 xyz/1
  Mux1/1 -> RotMat2AxisAngle/1(RotMat_Visu)  "RotationMatrix Visu"
  Fcn17/1 -> Mux1/9
  Fcn16/1 -> Mux1/8
  Fcn15/1 -> Mux1/7
  Fcn14/1 -> Mux1/6
  Fcn13/1 -> Mux1/5
  Fcn12/1 -> Mux1/4
  Fcn11/1 -> Mux1/3
  Fcn10/1 -> Mux1/2
  Fcn9/1 -> Mux1/1

== system ADAC_AEBS_FailOperationTest_A2_cs/VISUWheels_Citroen_C3_1/conv_RotWheelRL ==
  BryantISO [deg] : Inport
  Fcn10 : Fcn  Expr=cos(u(1))*sin(u(3))+sin(u(1))*sin(u(2))*cos(u(3))
  Fcn11 : Fcn  Expr=sin(u(1))*sin(u(3))-cos(u(1))*sin(u(2))*cos(u(3))
  Fcn12 : Fcn  Expr=-cos(u(2))*sin(u(3))
  Fcn13 : Fcn  Expr=cos(u(1))*cos(u(3))-sin(u(1))*sin(u(2))*sin(u(3))
  Fcn14 : Fcn  Expr=sin(u(1))*cos(u(3))+cos(u(1))*sin(u(2))*sin(u(3))
  Fcn15 : Fcn  Expr=sin(u(2))
  Fcn16 : Fcn  Expr=-sin(u(1))*cos(u(2))
  Fcn17 : Fcn  Expr=cos(u(1))*cos(u(2))
  Fcn9 : Fcn  Expr=cos(u(2))*cos(u(3))
  Mux1 : Mux  Inputs=9
  RotMat2AxisAngle : Subsystem
  deg2rad : Gain  Gain=pi/180
  xyz 2 zxy : Selector  InputPortWidth=3  IndexOptions=Index vector (dialog)  Indices=[3 1 2]  OutputSizes=1
  zxy 2 xyz : Selector  InputPortWidth=4  IndexOptions=Index vector (dialog)  Indices=[2 3 1 4]  OutputSizes=1
  QuaternionVisu [rad] : Outport
  wires:
  zxy 2 xyz/1 -> QuaternionVisu [rad]/1
  xyz 2 zxy/1 -> deg2rad/1
  deg2rad/1 -> Fcn17/1, Fcn16/1, Fcn15/1, Fcn14/1, Fcn13/1, Fcn12/1, Fcn11/1, Fcn10/1, Fcn9/1
  BryantISO [deg]/1 -> xyz 2 zxy/1  "BryantAngles rotx roty rotz Visu"
  RotMat2AxisAngle/1(Angles_Visu) -> zxy 2 xyz/1
  Mux1/1 -> RotMat2AxisAngle/1(RotMat_Visu)  "RotationMatrix Visu"
  Fcn17/1 -> Mux1/9
  Fcn16/1 -> Mux1/8
  Fcn15/1 -> Mux1/7
  Fcn14/1 -> Mux1/6
  Fcn13/1 -> Mux1/5
  Fcn12/1 -> Mux1/4
  Fcn11/1 -> Mux1/3
  Fcn10/1 -> Mux1/2
  Fcn9/1 -> Mux1/1

== system ADAC_AEBS_FailOperationTest_A2_cs/VISUWheels_Citroen_C3_1/conv_RotWheelRR ==
  BryantISO [deg] : Inport
  Fcn10 : Fcn  Expr=cos(u(1))*sin(u(3))+sin(u(1))*sin(u(2))*cos(u(3))
  Fcn11 : Fcn  Expr=sin(u(1))*sin(u(3))-cos(u(1))*sin(u(2))*cos(u(3))
  Fcn12 : Fcn  Expr=-cos(u(2))*sin(u(3))
  Fcn13 : Fcn  Expr=cos(u(1))*cos(u(3))-sin(u(1))*sin(u(2))*sin(u(3))
  Fcn14 : Fcn  Expr=sin(u(1))*cos(u(3))+cos(u(1))*sin(u(2))*sin(u(3))
  Fcn15 : Fcn  Expr=sin(u(2))
  Fcn16 : Fcn  Expr=-sin(u(1))*cos(u(2))
  Fcn17 : Fcn  Expr=cos(u(1))*cos(u(2))
  Fcn9 : Fcn  Expr=cos(u(2))*cos(u(3))
  Mux1 : Mux  Inputs=9
  RotMat2AxisAngle : Subsystem
  deg2rad : Gain  Gain=pi/180
  xyz 2 zxy : Selector  InputPortWidth=3  IndexOptions=Index vector (dialog)  Indices=[3 1 2]  OutputSizes=1
  zxy 2 xyz : Selector  InputPortWidth=4  IndexOptions=Index vector (dialog)  Indices=[2 3 1 4]  OutputSizes=1
  QuaternionVisu [rad] : Outport
  wires:
  zxy 2 xyz/1 -> QuaternionVisu [rad]/1
  xyz 2 zxy/1 -> deg2rad/1
  deg2rad/1 -> Fcn17/1, Fcn16/1, Fcn15/1, Fcn14/1, Fcn13/1, Fcn12/1, Fcn11/1, Fcn10/1, Fcn9/1
  BryantISO [deg]/1 -> xyz 2 zxy/1  "BryantAngles rotx roty rotz Visu"
  RotMat2AxisAngle/1(Angles_Visu) -> zxy 2 xyz/1
  Mux1/1 -> RotMat2AxisAngle/1(RotMat_Visu)  "RotationMatrix Visu"
  Fcn17/1 -> Mux1/9
  Fcn16/1 -> Mux1/8
  Fcn15/1 -> Mux1/7
  Fcn14/1 -> Mux1/6
  Fcn13/1 -> Mux1/5
  Fcn12/1 -> Mux1/4
  Fcn11/1 -> Mux1/3
  Fcn10/1 -> Mux1/2
  Fcn9/1 -> Mux1/1

== system ADAC_AEBS_FailOperationTest_A2_cs/VISUWheels_Citroen_C3_1/conv_TransWheelFL ==
  transISO [m] : Inport
  Gain1 : Gain  Gain=Gain_xISO
  Gain2 : Gain  Gain=Gain_yISO
  Gain3 : Gain  Gain=Gain_zISO
  Mux2 : Mux  Inputs=3
  Sum : Sum  Inputs=|++
  pos_ini_Visu : Subsystem
  transISO2Visu : Subsystem
  transVisu [m] : Outport
  wires:
  Gain3/1 -> Mux2/3
  Gain2/1 -> Mux2/2
  Gain1/1 -> Mux2/1
  Sum/1 -> transVisu [m]/1
  pos_ini_Visu/1(pos_ini_Visu) -> Sum/2
  Mux2/1 -> Sum/1
  transISO [m]/1 -> transISO2Visu/1(transISO)
  transISO2Visu/1(trans_x_Visu) -> Gain1/1
  transISO2Visu/2(trans_y_Visu) -> Gain2/1
  transISO2Visu/3(trans_z_Visu) -> Gain3/1

== system ADAC_AEBS_FailOperationTest_A2_cs/VISUWheels_Citroen_C3_1/conv_TransWheelFR ==
  transISO [m] : Inport
  Gain1 : Gain  Gain=Gain_xISO
  Gain2 : Gain  Gain=Gain_yISO
  Gain3 : Gain  Gain=Gain_zISO
  Mux2 : Mux  Inputs=3
  Sum : Sum  Inputs=|++
  pos_ini_Visu : Subsystem
  transISO2Visu : Subsystem
  transVisu [m] : Outport
  wires:
  Gain3/1 -> Mux2/3
  Gain2/1 -> Mux2/2
  Gain1/1 -> Mux2/1
  Sum/1 -> transVisu [m]/1
  pos_ini_Visu/1(pos_ini_Visu) -> Sum/2
  Mux2/1 -> Sum/1
  transISO [m]/1 -> transISO2Visu/1(transISO)
  transISO2Visu/1(trans_x_Visu) -> Gain1/1
  transISO2Visu/2(trans_y_Visu) -> Gain2/1
  transISO2Visu/3(trans_z_Visu) -> Gain3/1

== system ADAC_AEBS_FailOperationTest_A2_cs/VISUWheels_Citroen_C3_1/conv_TransWheelRL ==
  transISO [m] : Inport
  Gain1 : Gain  Gain=Gain_xISO
  Gain2 : Gain  Gain=Gain_yISO
  Gain3 : Gain  Gain=Gain_zISO
  Mux2 : Mux  Inputs=3
  Sum : Sum  Inputs=|++
  pos_ini_Visu : Subsystem
  transISO2Visu : Subsystem
  transVisu [m] : Outport
  wires:
  Gain3/1 -> Mux2/3
  Gain2/1 -> Mux2/2
  Gain1/1 -> Mux2/1
  Sum/1 -> transVisu [m]/1
  pos_ini_Visu/1(pos_ini_Visu) -> Sum/2
  Mux2/1 -> Sum/1
  transISO2Visu/3(trans_z_Visu) -> Gain3/1
  transISO2Visu/2(trans_y_Visu) -> Gain2/1
  transISO [m]/1 -> transISO2Visu/1(transISO)
  transISO2Visu/1(trans_x_Visu) -> Gain1/1

== system ADAC_AEBS_FailOperationTest_A2_cs/VISUWheels_Citroen_C3_1/conv_TransWheelRR ==
  transISO [m] : Inport
  Gain1 : Gain  Gain=Gain_xISO
  Gain2 : Gain  Gain=Gain_yISO
  Gain3 : Gain  Gain=Gain_zISO
  Mux2 : Mux  Inputs=3
  Sum : Sum  Inputs=|++
  pos_ini_Visu : Subsystem
  transISO2Visu : Subsystem
  transVisu [m] : Outport
  wires:
  Gain3/1 -> Mux2/3
  Gain2/1 -> Mux2/2
  Gain1/1 -> Mux2/1
  Sum/1 -> transVisu [m]/1
  pos_ini_Visu/1(pos_ini_Visu) -> Sum/2
  Mux2/1 -> Sum/1
  transISO2Visu/3(trans_z_Visu) -> Gain3/1
  transISO2Visu/2(trans_y_Visu) -> Gain2/1
  transISO [m]/1 -> transISO2Visu/1(transISO)
  transISO2Visu/1(trans_x_Visu) -> Gain1/1

== system ADAC_AEBS_FailOperationTest_A2_cs/VISUWheels_Citroen_C3_1/visu_RotWheelFL ==
  Y : Inport
  Assignment : Assignment  IndexMode=Zero-based  SampleTime=TimeStep  IndexOptions=Starting index (dialog)  Indices=PortIndex  OutputSizes=[1 1]
  Data Store Read : DataStoreRead  DataStoreName=SimCoreActuators  SampleTime=TimeStep
  Data Store Write : DataStoreWrite  DataStoreName=SimCoreActuators
  wires:
  Y/1 -> Assignment/2
  Data Store Read/1 -> Assignment/1
  Assignment/1 -> Data Store Write/1

== system ADAC_AEBS_FailOperationTest_A2_cs/VISUWheels_Citroen_C3_1/visu_RotWheelFR ==
  Y : Inport
  Assignment : Assignment  IndexMode=Zero-based  SampleTime=TimeStep  IndexOptions=Starting index (dialog)  Indices=PortIndex  OutputSizes=[1 1]
  Data Store Read : DataStoreRead  DataStoreName=SimCoreActuators  SampleTime=TimeStep
  Data Store Write : DataStoreWrite  DataStoreName=SimCoreActuators
  wires:
  Y/1 -> Assignment/2
  Data Store Read/1 -> Assignment/1
  Assignment/1 -> Data Store Write/1

== system ADAC_AEBS_FailOperationTest_A2_cs/VISUWheels_Citroen_C3_1/visu_RotWheelRL ==
  Y : Inport
  Assignment : Assignment  IndexMode=Zero-based  SampleTime=TimeStep  IndexOptions=Starting index (dialog)  Indices=PortIndex  OutputSizes=[1 1]
  Data Store Read : DataStoreRead  DataStoreName=SimCoreActuators  SampleTime=TimeStep
  Data Store Write : DataStoreWrite  DataStoreName=SimCoreActuators
  wires:
  Y/1 -> Assignment/2
  Data Store Read/1 -> Assignment/1
  Assignment/1 -> Data Store Write/1

== system ADAC_AEBS_FailOperationTest_A2_cs/VISUWheels_Citroen_C3_1/visu_RotWheelRR ==
  Y : Inport
  Assignment : Assignment  IndexMode=Zero-based  SampleTime=TimeStep  IndexOptions=Starting index (dialog)  Indices=PortIndex  OutputSizes=[1 1]
  Data Store Read : DataStoreRead  DataStoreName=SimCoreActuators  SampleTime=TimeStep
  Data Store Write : DataStoreWrite  DataStoreName=SimCoreActuators
  wires:
  Y/1 -> Assignment/2
  Data Store Read/1 -> Assignment/1
  Assignment/1 -> Data Store Write/1

== system ADAC_AEBS_FailOperationTest_A2_cs/VISUWheels_Citroen_C3_1/visu_TransWheelFL ==
  Y : Inport
  Assignment : Assignment  IndexMode=Zero-based  SampleTime=TimeStep  IndexOptions=Starting index (dialog)  Indices=PortIndex  OutputSizes=[1 1]
  Data Store Read : DataStoreRead  DataStoreName=SimCoreActuators  SampleTime=TimeStep
  Data Store Write : DataStoreWrite  DataStoreName=SimCoreActuators
  wires:
  Y/1 -> Assignment/2
  Data Store Read/1 -> Assignment/1
  Assignment/1 -> Data Store Write/1
